simulink model "simulink_execution"  (R2021a)
settings: Solver=ode45  StartTime=0.0  StopTime=20.0  RelTol=1e-3
libraries: simulink x2
settings Model: EnablePacing=on  Creator=sprinkle  LastModifiedBy=sprinkle

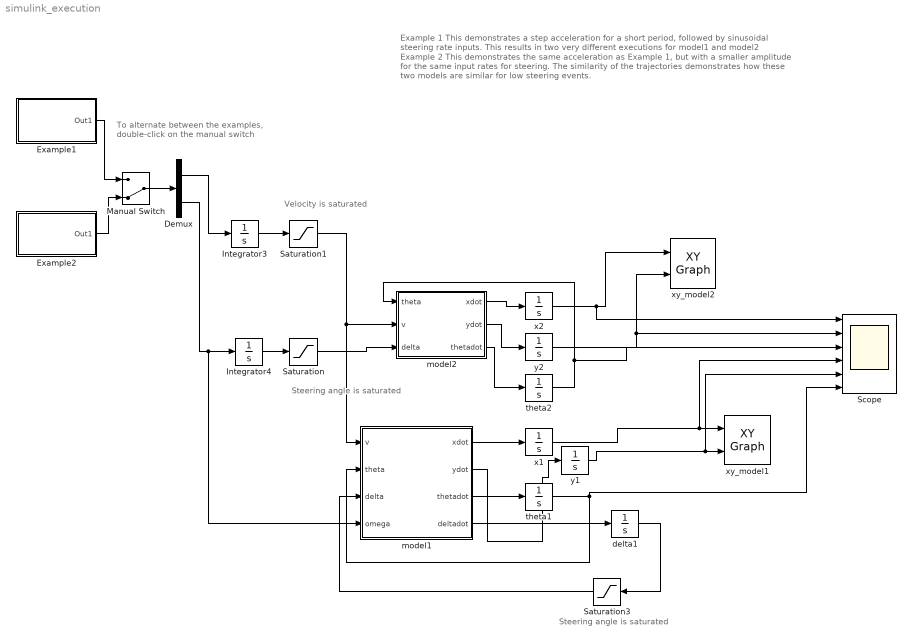
== system simulink_execution ==
  note: Steering angle is saturated
  note: To alternate between the examples, double-click on the manual switch
  note: Example 1
      |
      | This demonstrates a step acceleration for a short period, followed by sinusoidal steering rate inputs. This results in two very different executions for model1 and model2
      |
      | Example 2
      |
      | This demonstrates the same acceleration as Example 1, but with a smaller amplitude for the same input rates for steering. The similarity of the trajectories demonstrates how these two models are similar for low steering events.
  note: Velocity is saturated
  note: Steering angle is saturated
  Demux : Demux  Outputs=2
  Example1 : Subsystem
  Example2 : Subsystem
  Integrator3 : Integrator
  Integrator4 : Integrator
  Manual Switch : ManualSwitch  CurrentSetting=0
  Saturation : Saturate  UpperLimit=pi/6  LowerLimit=-pi/6
  Saturation1 : Saturate  UpperLimit=5  LowerLimit=0
  Saturation3 : Saturate  UpperLimit=pi/6  LowerLimit=-pi/6
  Scope : Scope  NumInputPorts=6
  delta1 : Integrator
  model1 : MATLAB Function  TreatAsAtomicUnit=on
  model2 : MATLAB Function  TreatAsAtomicUnit=on
  theta1 : Integrator
  theta2 : Integrator
  x1 : Integrator
  x2 : Integrator
  xy_model1 : simulink/Sinks/XY Graph  xmin=-30  xmax=30  ymin=-30  ymax=30  st=-1
  xy_model2 : simulink/Sinks/XY Graph  xmin=-30  xmax=30  ymin=-30  ymax=30  st=-1
  y1 : Integrator
  y2 : Integrator
  wires:
  model2/1(xdot) -> x2/1
  model2/2(ydot) -> y2/1
  model2/3(thetadot) -> theta2/1
  theta2/1 -> Scope/3, model2/1(theta)
  Integrator3/1 -> Saturation1/1
  Integrator4/1 -> Saturation/1
  x2/1 -> Scope/1, xy_model2/1
  y2/1 -> Scope/2, xy_model2/2
  Saturation/1 -> model2/3(delta)
  Saturation1/1 -> model1/1(v), model2/2(v)
  model1/1(xdot) -> x1/1
  model1/2(ydot) -> y1/1
  model1/3(thetadot) -> theta1/1
  model1/4(deltadot) -> delta1/1
  theta1/1 -> model1/2(theta), Scope/6
  delta1/1 -> Saturation3/1
  x1/1 -> Scope/4, xy_model1/1
  y1/1 -> Scope/5, xy_model1/2
  Saturation3/1 -> model1/3(delta)
  Demux/2 -> model1/4(omega), Integrator4/1
  Demux/1 -> Integrator3/1
  Manual Switch/1 -> Demux/1
  Example1/1(Out1) -> Manual Switch/1
  Example2/1(Out1) -> Manual Switch/2

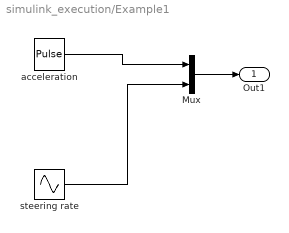
== system simulink_execution/Example1 ==
  Mux : Mux  Inputs=2
  acceleration : DiscretePulseGenerator  PulseType=Time based  Amplitude=1.0  Period=20  PulseWidth=50
  steering rate : Sin  Amplitude=0.5  SampleTime=0
  Out1 : Outport
  wires:
  acceleration/1 -> Mux/1
  steering rate/1 -> Mux/2
  Mux/1 -> Out1/1

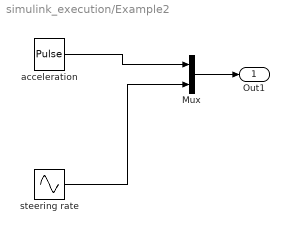
== system simulink_execution/Example2 ==
  Mux : Mux  Inputs=2
  acceleration : DiscretePulseGenerator  PulseType=Time based  Amplitude=1.0  Period=20  PulseWidth=50
  steering rate : Sin  Amplitude=0.05  SampleTime=0
  Out1 : Outport
  wires:
  acceleration/1 -> Mux/1
  steering rate/1 -> Mux/2
  Mux/1 -> Out1/1

== matlab function simulink_execution/model1 ==
  data: v input; xdot output; theta input; delta input; omega input; ydot output; thetadot output; deltadot output
function [xdot, ydot, thetadot, deltadot] = fcn(v,theta,delta,omega)

% L is the wheelbase, and is a constant
L = 2.62;

% the deltaT term is taken care of in simulink integration now
xdot = v*cos(theta)*cos(delta);
ydot = v*sin(theta)*cos(delta);
thetadot = (v/L)*sin(delta);
deltadot = omega;

end

== matlab function simulink_execution/model2 ==
  data: theta input; xdot output; v input; delta input; ydot output; thetadot output
function [xdot, ydot, thetadot] = fcn(theta,v,delta)

% L is the wheelbase of the vehicle (distance from the center of the front
% two tires to the center of the rear two tires) and is a constant
L = 2.62; % in meters

% the simulink version does not include a deltaT term, but is integrated
% after the block
xdot     = v*cos(theta);
ydot     = v*sin(theta);
thetadot = v*(tan(delta)/L);

end
